simulink library "mylib"  (R2020a)
settings: Solver=VariableStepAuto  StartTime=0.0  StopTime=10.0  RelTol=1e-3
undefined symbols (not defined in the file): d_du_max_pu, dir_to_bus1, dir_to_bus_0L, dir_to_bus_2, dir_to_line1, dir_to_line_0L, dir_to_line_2, du_max_pu, du_ph_max_pu, Fi_0, Fi_T_H, Fi_T_L, Fi_T_M, I0_calc_0L, I0_comp_H, I0_comp_L, I0_comp_M, I0_max_0L, I2_max_2, I_diff1, I_diff2, I_diff3, I_diff4, I_diff5, I_diff_to, I_hight_CT1_G, I_hight_CT2_G, I_low_CT1, I_low_CT2, I_max1, I_max2, I_max3, I_max4, I_max5, I_min_sec_CT1, I_min_sec_CT2, I_unb, Iph_max_0L, Iph_max_2, jmp_in_zone, jmp_in_zone_0L, jmp_in_zone_2, K_dop, max_min1, only_K1_0L, only_K1_2, only_K2_0L, only_K2_2, only_K3_0L, only_K3_2, P_ctl_0, PQ_Fi_ctl_0, Q_ctl_0, S_set_0, set, set1, T_fast, T_I_ctl, T_off, T_on ... (+15)
libraries: $bdroot x184, powerlib_meascontrol x97
(part 12 of 14)

== system mylib/278_dzt_v1/diff_brake/calc_brake_Ia/cut_brake_1 ==
  Y_in : Inport
  I_max : Inport  Port=2
  I_diff_cur1 : Inport  Port=3
  I_max_cur1 : Inport  Port=4
  I_diff_cur2 : Inport  Port=5
  I_max_cur2 : Inport  Port=6
  I_diff_next : Inport  Port=7
  I_max_next : Inport  Port=8
  I_diff_to : Inport  Port=9
  1 : RelationalOperator  Operator=>  OutDataTypeStr=boolean  RndMeth=Simplest
  10 : Sum  Inputs=+-
  11 : Sum
  12 : Product
  13 : Sum
  {2,14..16,20} (5 alike) : Switch  Criteria=u2 > Threshold
  157 : Constant  Value=0
  17 : Logic  AllPortsSameDT=off  OutDataTypeStr=boolean
  18 : Logic  AllPortsSameDT=off  OutDataTypeStr=boolean
  19 : Logic  Operator=NOT  AllPortsSameDT=off  OutDataTypeStr=boolean
  3 : Product  Inputs=*/  RndMeth=Zero  SaturateOnIntegerOverflow=on
  4 : Product
  5 : Sum
  6 : RelationalOperator  Operator=<=  OutDataTypeStr=boolean  RndMeth=Simplest
  7 : RelationalOperator  Operator=>  OutDataTypeStr=boolean  RndMeth=Simplest
  8 : Logic  Operator=OR  AllPortsSameDT=off  OutDataTypeStr=boolean
  9 : RelationalOperator  Operator===  OutDataTypeStr=boolean  RndMeth=Simplest
  ADD_B : Subsystem
  ADD_K : Subsystem
  z_ch : Subsystem
  z_ch1 : Subsystem
  z_ch2 : Subsystem
  I_brake : Outport
  wires:
  20/1 -> 7/2, 6/2
  11/1 -> 20/1
  18/1 -> 20/2
  z_ch2/1(out) -> 18/1
  19/1 -> 18/2
  5/1 -> 2/1
  17/1 -> 2/2
  6/1 -> 17/2
  1/1 -> 17/1
  7/1 -> 15/2
  4/1 -> 5/1
  2/1 -> 15/3
  14/1 -> 15/1
  8/1 -> 16/2
  15/1 -> 16/3
  16/1 -> I_brake/1
  9/1 -> 19/1, 14/2
  13/1 -> 14/1
  ADD_B/1(out) -> 13/2, 5/2
  12/1 -> 13/1
  157/1 -> 9/2
  I_diff_to/1 -> 10/1, 14/3, 9/1
  3/1 -> 11/1
  10/1 -> 3/1
  ADD_K/1(out) -> 3/2, 12/1, 4/2
  I_max_next/1 -> z_ch2/2(in2)
  I_diff_next/1 -> z_ch2/1(in1)
  I_max_cur2/1 -> z_ch1/2(in2), ADD_B/2(X2), ADD_K/3(X2), 20/3
  I_diff_cur2/1 -> ADD_B/3(Y2), ADD_K/1(Y2), z_ch1/1(in1)
  I_max_cur1/1 -> ADD_B/4(X1), ADD_K/4(X1), 1/2, z_ch/2(in2), 11/2
  I_diff_cur1/1 -> z_ch/1(in1), ADD_B/1(Y1), ADD_K/2(Y1), 10/2
  z_ch1/1(out) -> 8/2
  z_ch/1(out) -> 8/1
  I_max/1 -> 1/1, 6/1, 4/1, 7/1, 12/2
  Y_in/1 -> 2/3, 16/1

== system mylib/278_dzt_v1/diff_brake/calc_brake_Ia/cut_brake_2 ==
  Y_in : Inport
  I_max : Inport  Port=2
  I_diff_cur1 : Inport  Port=3
  I_max_cur1 : Inport  Port=4
  I_diff_cur2 : Inport  Port=5
  I_max_cur2 : Inport  Port=6
  I_diff_next : Inport  Port=7
  I_max_next : Inport  Port=8
  I_diff_to : Inport  Port=9
  1 : RelationalOperator  Operator=>  OutDataTypeStr=boolean  RndMeth=Simplest
  10 : Sum  Inputs=+-
  11 : Sum
  12 : Product
  13 : Sum
  {2,14..16,20} (5 alike) : Switch  Criteria=u2 > Threshold
  157 : Constant  Value=0
  17 : Logic  AllPortsSameDT=off  OutDataTypeStr=boolean
  18 : Logic  AllPortsSameDT=off  OutDataTypeStr=boolean
  19 : Logic  Operator=NOT  AllPortsSameDT=off  OutDataTypeStr=boolean
  3 : Product  Inputs=*/  RndMeth=Zero  SaturateOnIntegerOverflow=on
  4 : Product
  5 : Sum
  6 : RelationalOperator  Operator=<=  OutDataTypeStr=boolean  RndMeth=Simplest
  7 : RelationalOperator  Operator=>  OutDataTypeStr=boolean  RndMeth=Simplest
  8 : Logic  Operator=OR  AllPortsSameDT=off  OutDataTypeStr=boolean
  9 : RelationalOperator  Operator===  OutDataTypeStr=boolean  RndMeth=Simplest
  ADD_B : Subsystem
  ADD_K : Subsystem
  z_ch : Subsystem
  z_ch1 : Subsystem
  z_ch2 : Subsystem
  I_brake : Outport
  wires:
  20/1 -> 7/2, 6/2
  11/1 -> 20/1
  18/1 -> 20/2
  z_ch2/1(out) -> 18/1
  19/1 -> 18/2
  5/1 -> 2/1
  17/1 -> 2/2
  6/1 -> 17/2
  1/1 -> 17/1
  7/1 -> 15/2
  4/1 -> 5/1
  2/1 -> 15/3
  14/1 -> 15/1
  8/1 -> 16/2
  15/1 -> 16/3
  16/1 -> I_brake/1
  9/1 -> 19/1, 14/2
  13/1 -> 14/1
  ADD_B/1(out) -> 13/2, 5/2
  12/1 -> 13/1
  157/1 -> 9/2
  I_diff_to/1 -> 10/1, 14/3, 9/1
  3/1 -> 11/1
  10/1 -> 3/1
  ADD_K/1(out) -> 3/2, 12/1, 4/2
  I_max_next/1 -> z_ch2/2(in2)
  I_diff_next/1 -> z_ch2/1(in1)
  I_max_cur2/1 -> z_ch1/2(in2), ADD_B/2(X2), ADD_K/3(X2), 20/3
  I_diff_cur2/1 -> ADD_B/3(Y2), ADD_K/1(Y2), z_ch1/1(in1)
  I_max_cur1/1 -> ADD_B/4(X1), ADD_K/4(X1), 1/2, z_ch/2(in2), 11/2
  I_diff_cur1/1 -> z_ch/1(in1), ADD_B/1(Y1), ADD_K/2(Y1), 10/2
  z_ch1/1(out) -> 8/2
  z_ch/1(out) -> 8/1
  I_max/1 -> 1/1, 6/1, 4/1, 7/1, 12/2
  Y_in/1 -> 2/3, 16/1

== system mylib/278_dzt_v1/diff_brake/calc_brake_Ia/cut_brake_3 ==
  Y_in : Inport
  I_max : Inport  Port=2
  I_diff_cur1 : Inport  Port=3
  I_max_cur1 : Inport  Port=4
  I_diff_cur2 : Inport  Port=5
  I_max_cur2 : Inport  Port=6
  I_diff_next : Inport  Port=7
  I_max_next : Inport  Port=8
  I_diff_to : Inport  Port=9
  1 : RelationalOperator  Operator=>  OutDataTypeStr=boolean  RndMeth=Simplest
  10 : Sum  Inputs=+-
  11 : Sum
  12 : Product
  13 : Sum
  {2,14..16,20} (5 alike) : Switch  Criteria=u2 > Threshold
  157 : Constant  Value=0
  17 : Logic  AllPortsSameDT=off  OutDataTypeStr=boolean
  18 : Logic  AllPortsSameDT=off  OutDataTypeStr=boolean
  19 : Logic  Operator=NOT  AllPortsSameDT=off  OutDataTypeStr=boolean
  3 : Product  Inputs=*/  RndMeth=Zero  SaturateOnIntegerOverflow=on
  4 : Product
  5 : Sum
  6 : RelationalOperator  Operator=<=  OutDataTypeStr=boolean  RndMeth=Simplest
  7 : RelationalOperator  Operator=>  OutDataTypeStr=boolean  RndMeth=Simplest
  8 : Logic  Operator=OR  AllPortsSameDT=off  OutDataTypeStr=boolean
  9 : RelationalOperator  Operator===  OutDataTypeStr=boolean  RndMeth=Simplest
  ADD_B : Subsystem
  ADD_K : Subsystem
  z_ch : Subsystem
  z_ch1 : Subsystem
  z_ch2 : Subsystem
  I_brake : Outport
  wires:
  20/1 -> 7/2, 6/2
  11/1 -> 20/1
  18/1 -> 20/2
  z_ch2/1(out) -> 18/1
  19/1 -> 18/2
  5/1 -> 2/1
  17/1 -> 2/2
  6/1 -> 17/2
  1/1 -> 17/1
  7/1 -> 15/2
  4/1 -> 5/1
  2/1 -> 15/3
  14/1 -> 15/1
  8/1 -> 16/2
  15/1 -> 16/3
  16/1 -> I_brake/1
  9/1 -> 19/1, 14/2
  13/1 -> 14/1
  ADD_B/1(out) -> 13/2, 5/2
  12/1 -> 13/1
  157/1 -> 9/2
  I_diff_to/1 -> 10/1, 14/3, 9/1
  3/1 -> 11/1
  10/1 -> 3/1
  ADD_K/1(out) -> 3/2, 12/1, 4/2
  I_max_next/1 -> z_ch2/2(in2)
  I_diff_next/1 -> z_ch2/1(in1)
  I_max_cur2/1 -> z_ch1/2(in2), ADD_B/2(X2), ADD_K/3(X2), 20/3
  I_diff_cur2/1 -> ADD_B/3(Y2), ADD_K/1(Y2), z_ch1/1(in1)
  I_max_cur1/1 -> ADD_B/4(X1), ADD_K/4(X1), 1/2, z_ch/2(in2), 11/2
  I_diff_cur1/1 -> z_ch/1(in1), ADD_B/1(Y1), ADD_K/2(Y1), 10/2
  z_ch1/1(out) -> 8/2
  z_ch/1(out) -> 8/1
  I_max/1 -> 1/1, 6/1, 4/1, 7/1, 12/2
  Y_in/1 -> 2/3, 16/1

== system mylib/278_dzt_v1/diff_brake/calc_brake_Ia/cut_brake_4 ==
  Y_in : Inport
  I_max : Inport  Port=2
  I_diff_cur1 : Inport  Port=3
  I_max_cur1 : Inport  Port=4
  I_diff_cur2 : Inport  Port=5
  I_max_cur2 : Inport  Port=6
  I_diff_next : Inport  Port=7
  I_max_next : Inport  Port=8
  I_diff_to : Inport  Port=9
  1 : RelationalOperator  Operator=>  OutDataTypeStr=boolean  RndMeth=Simplest
  10 : Sum  Inputs=+-
  11 : Sum
  12 : Product
  13 : Sum
  {2,14..16,20} (5 alike) : Switch  Criteria=u2 > Threshold
  157 : Constant  Value=0
  17 : Logic  AllPortsSameDT=off  OutDataTypeStr=boolean
  18 : Logic  AllPortsSameDT=off  OutDataTypeStr=boolean
  19 : Logic  Operator=NOT  AllPortsSameDT=off  OutDataTypeStr=boolean
  3 : Product  Inputs=*/  RndMeth=Zero  SaturateOnIntegerOverflow=on
  4 : Product
  5 : Sum
  6 : RelationalOperator  Operator=<=  OutDataTypeStr=boolean  RndMeth=Simplest
  7 : RelationalOperator  Operator=>  OutDataTypeStr=boolean  RndMeth=Simplest
  8 : Logic  Operator=OR  AllPortsSameDT=off  OutDataTypeStr=boolean
  9 : RelationalOperator  Operator===  OutDataTypeStr=boolean  RndMeth=Simplest
  ADD_B : Subsystem
  ADD_K : Subsystem
  z_ch : Subsystem
  z_ch1 : Subsystem
  z_ch2 : Subsystem
  I_brake : Outport
  wires:
  20/1 -> 7/2, 6/2
  11/1 -> 20/1
  18/1 -> 20/2
  z_ch2/1(out) -> 18/1
  19/1 -> 18/2
  5/1 -> 2/1
  17/1 -> 2/2
  6/1 -> 17/2
  1/1 -> 17/1
  7/1 -> 15/2
  4/1 -> 5/1
  2/1 -> 15/3
  14/1 -> 15/1
  8/1 -> 16/2
  15/1 -> 16/3
  16/1 -> I_brake/1
  9/1 -> 19/1, 14/2
  13/1 -> 14/1
  ADD_B/1(out) -> 13/2, 5/2
  12/1 -> 13/1
  157/1 -> 9/2
  I_diff_to/1 -> 10/1, 14/3, 9/1
  3/1 -> 11/1
  10/1 -> 3/1
  ADD_K/1(out) -> 3/2, 12/1, 4/2
  I_max_next/1 -> z_ch2/2(in2)
  I_diff_next/1 -> z_ch2/1(in1)
  I_max_cur2/1 -> z_ch1/2(in2), ADD_B/2(X2), ADD_K/3(X2), 20/3
  I_diff_cur2/1 -> ADD_B/3(Y2), ADD_K/1(Y2), z_ch1/1(in1)
  I_max_cur1/1 -> ADD_B/4(X1), ADD_K/4(X1), 1/2, z_ch/2(in2), 11/2
  I_diff_cur1/1 -> z_ch/1(in1), ADD_B/1(Y1), ADD_K/2(Y1), 10/2
  z_ch1/1(out) -> 8/2
  z_ch/1(out) -> 8/1
  I_max/1 -> 1/1, 6/1, 4/1, 7/1, 12/2
  Y_in/1 -> 2/3, 16/1

== system mylib/278_dzt_v1/diff_brake/calc_brake_Ib/cut_brake_1 ==
  Y_in : Inport
  I_max : Inport  Port=2
  I_diff_cur1 : Inport  Port=3
  I_max_cur1 : Inport  Port=4
  I_diff_cur2 : Inport  Port=5
  I_max_cur2 : Inport  Port=6
  I_diff_next : Inport  Port=7
  I_max_next : Inport  Port=8
  I_diff_to : Inport  Port=9
  1 : RelationalOperator  Operator=>  OutDataTypeStr=boolean  RndMeth=Simplest
  10 : Sum  Inputs=+-
  11 : Sum
  12 : Product
  13 : Sum
  {2,14..16,20} (5 alike) : Switch  Criteria=u2 > Threshold
  157 : Constant  Value=0
  17 : Logic  AllPortsSameDT=off  OutDataTypeStr=boolean
  18 : Logic  AllPortsSameDT=off  OutDataTypeStr=boolean
  19 : Logic  Operator=NOT  AllPortsSameDT=off  OutDataTypeStr=boolean
  3 : Product  Inputs=*/  RndMeth=Zero  SaturateOnIntegerOverflow=on
  4 : Product
  5 : Sum
  6 : RelationalOperator  Operator=<=  OutDataTypeStr=boolean  RndMeth=Simplest
  7 : RelationalOperator  Operator=>  OutDataTypeStr=boolean  RndMeth=Simplest
  8 : Logic  Operator=OR  AllPortsSameDT=off  OutDataTypeStr=boolean
  9 : RelationalOperator  Operator===  OutDataTypeStr=boolean  RndMeth=Simplest
  ADD_B : Subsystem
  ADD_K : Subsystem
  z_ch : Subsystem
  z_ch1 : Subsystem
  z_ch2 : Subsystem
  I_brake : Outport
  wires:
  20/1 -> 7/2, 6/2
  11/1 -> 20/1
  18/1 -> 20/2
  z_ch2/1(out) -> 18/1
  19/1 -> 18/2
  5/1 -> 2/1
  17/1 -> 2/2
  6/1 -> 17/2
  1/1 -> 17/1
  7/1 -> 15/2
  4/1 -> 5/1
  2/1 -> 15/3
  14/1 -> 15/1
  8/1 -> 16/2
  15/1 -> 16/3
  16/1 -> I_brake/1
  9/1 -> 19/1, 14/2
  13/1 -> 14/1
  ADD_B/1(out) -> 13/2, 5/2
  12/1 -> 13/1
  157/1 -> 9/2
  I_diff_to/1 -> 10/1, 14/3, 9/1
  3/1 -> 11/1
  10/1 -> 3/1
  ADD_K/1(out) -> 3/2, 12/1, 4/2
  I_max_next/1 -> z_ch2/2(in2)
  I_diff_next/1 -> z_ch2/1(in1)
  I_max_cur2/1 -> z_ch1/2(in2), ADD_B/2(X2), ADD_K/3(X2), 20/3
  I_diff_cur2/1 -> ADD_B/3(Y2), ADD_K/1(Y2), z_ch1/1(in1)
  I_max_cur1/1 -> ADD_B/4(X1), ADD_K/4(X1), 1/2, z_ch/2(in2), 11/2
  I_diff_cur1/1 -> z_ch/1(in1), ADD_B/1(Y1), ADD_K/2(Y1), 10/2
  z_ch1/1(out) -> 8/2
  z_ch/1(out) -> 8/1
  I_max/1 -> 1/1, 6/1, 4/1, 7/1, 12/2
  Y_in/1 -> 2/3, 16/1

== system mylib/278_dzt_v1/diff_brake/calc_brake_Ib/cut_brake_2 ==
  Y_in : Inport
  I_max : Inport  Port=2
  I_diff_cur1 : Inport  Port=3
  I_max_cur1 : Inport  Port=4
  I_diff_cur2 : Inport  Port=5
  I_max_cur2 : Inport  Port=6
  I_diff_next : Inport  Port=7
  I_max_next : Inport  Port=8
  I_diff_to : Inport  Port=9
  1 : RelationalOperator  Operator=>  OutDataTypeStr=boolean  RndMeth=Simplest
  10 : Sum  Inputs=+-
  11 : Sum
  12 : Product
  13 : Sum
  {2,14..16,20} (5 alike) : Switch  Criteria=u2 > Threshold
  157 : Constant  Value=0
  17 : Logic  AllPortsSameDT=off  OutDataTypeStr=boolean
  18 : Logic  AllPortsSameDT=off  OutDataTypeStr=boolean
  19 : Logic  Operator=NOT  AllPortsSameDT=off  OutDataTypeStr=boolean
  3 : Product  Inputs=*/  RndMeth=Zero  SaturateOnIntegerOverflow=on
  4 : Product
  5 : Sum
  6 : RelationalOperator  Operator=<=  OutDataTypeStr=boolean  RndMeth=Simplest
  7 : RelationalOperator  Operator=>  OutDataTypeStr=boolean  RndMeth=Simplest
  8 : Logic  Operator=OR  AllPortsSameDT=off  OutDataTypeStr=boolean
  9 : RelationalOperator  Operator===  OutDataTypeStr=boolean  RndMeth=Simplest
  ADD_B : Subsystem
  ADD_K : Subsystem
  z_ch : Subsystem
  z_ch1 : Subsystem
  z_ch2 : Subsystem
  I_brake : Outport
  wires:
  20/1 -> 7/2, 6/2
  11/1 -> 20/1
  18/1 -> 20/2
  z_ch2/1(out) -> 18/1
  19/1 -> 18/2
  5/1 -> 2/1
  17/1 -> 2/2
  6/1 -> 17/2
  1/1 -> 17/1
  7/1 -> 15/2
  4/1 -> 5/1
  2/1 -> 15/3
  14/1 -> 15/1
  8/1 -> 16/2
  15/1 -> 16/3
  16/1 -> I_brake/1
  9/1 -> 19/1, 14/2
  13/1 -> 14/1
  ADD_B/1(out) -> 13/2, 5/2
  12/1 -> 13/1
  157/1 -> 9/2
  I_diff_to/1 -> 10/1, 14/3, 9/1
  3/1 -> 11/1
  10/1 -> 3/1
  ADD_K/1(out) -> 3/2, 12/1, 4/2
  I_max_next/1 -> z_ch2/2(in2)
  I_diff_next/1 -> z_ch2/1(in1)
  I_max_cur2/1 -> z_ch1/2(in2), ADD_B/2(X2), ADD_K/3(X2), 20/3
  I_diff_cur2/1 -> ADD_B/3(Y2), ADD_K/1(Y2), z_ch1/1(in1)
  I_max_cur1/1 -> ADD_B/4(X1), ADD_K/4(X1), 1/2, z_ch/2(in2), 11/2
  I_diff_cur1/1 -> z_ch/1(in1), ADD_B/1(Y1), ADD_K/2(Y1), 10/2
  z_ch1/1(out) -> 8/2
  z_ch/1(out) -> 8/1
  I_max/1 -> 1/1, 6/1, 4/1, 7/1, 12/2
  Y_in/1 -> 2/3, 16/1

== system mylib/278_dzt_v1/diff_brake/calc_brake_Ib/cut_brake_3 ==
  Y_in : Inport
  I_max : Inport  Port=2
  I_diff_cur1 : Inport  Port=3
  I_max_cur1 : Inport  Port=4
  I_diff_cur2 : Inport  Port=5
  I_max_cur2 : Inport  Port=6
  I_diff_next : Inport  Port=7
  I_max_next : Inport  Port=8
  I_diff_to : Inport  Port=9
  1 : RelationalOperator  Operator=>  OutDataTypeStr=boolean  RndMeth=Simplest
  10 : Sum  Inputs=+-
  11 : Sum
  12 : Product
  13 : Sum
  {2,14..16,20} (5 alike) : Switch  Criteria=u2 > Threshold
  157 : Constant  Value=0
  17 : Logic  AllPortsSameDT=off  OutDataTypeStr=boolean
  18 : Logic  AllPortsSameDT=off  OutDataTypeStr=boolean
  19 : Logic  Operator=NOT  AllPortsSameDT=off  OutDataTypeStr=boolean
  3 : Product  Inputs=*/  RndMeth=Zero  SaturateOnIntegerOverflow=on
  4 : Product
  5 : Sum
  6 : RelationalOperator  Operator=<=  OutDataTypeStr=boolean  RndMeth=Simplest
  7 : RelationalOperator  Operator=>  OutDataTypeStr=boolean  RndMeth=Simplest
  8 : Logic  Operator=OR  AllPortsSameDT=off  OutDataTypeStr=boolean
  9 : RelationalOperator  Operator===  OutDataTypeStr=boolean  RndMeth=Simplest
  ADD_B : Subsystem
  ADD_K : Subsystem
  z_ch : Subsystem
  z_ch1 : Subsystem
  z_ch2 : Subsystem
  I_brake : Outport
  wires:
  20/1 -> 7/2, 6/2
  11/1 -> 20/1
  18/1 -> 20/2
  z_ch2/1(out) -> 18/1
  19/1 -> 18/2
  5/1 -> 2/1
  17/1 -> 2/2
  6/1 -> 17/2
  1/1 -> 17/1
  7/1 -> 15/2
  4/1 -> 5/1
  2/1 -> 15/3
  14/1 -> 15/1
  8/1 -> 16/2
  15/1 -> 16/3
  16/1 -> I_brake/1
  9/1 -> 19/1, 14/2
  13/1 -> 14/1
  ADD_B/1(out) -> 13/2, 5/2
  12/1 -> 13/1
  157/1 -> 9/2
  I_diff_to/1 -> 10/1, 14/3, 9/1
  3/1 -> 11/1
  10/1 -> 3/1
  ADD_K/1(out) -> 3/2, 12/1, 4/2
  I_max_next/1 -> z_ch2/2(in2)
  I_diff_next/1 -> z_ch2/1(in1)
  I_max_cur2/1 -> z_ch1/2(in2), ADD_B/2(X2), ADD_K/3(X2), 20/3
  I_diff_cur2/1 -> ADD_B/3(Y2), ADD_K/1(Y2), z_ch1/1(in1)
  I_max_cur1/1 -> ADD_B/4(X1), ADD_K/4(X1), 1/2, z_ch/2(in2), 11/2
  I_diff_cur1/1 -> z_ch/1(in1), ADD_B/1(Y1), ADD_K/2(Y1), 10/2
  z_ch1/1(out) -> 8/2
  z_ch/1(out) -> 8/1
  I_max/1 -> 1/1, 6/1, 4/1, 7/1, 12/2
  Y_in/1 -> 2/3, 16/1

== system mylib/278_dzt_v1/diff_brake/calc_brake_Ib/cut_brake_4 ==
  Y_in : Inport
  I_max : Inport  Port=2
  I_diff_cur1 : Inport  Port=3
  I_max_cur1 : Inport  Port=4
  I_diff_cur2 : Inport  Port=5
  I_max_cur2 : Inport  Port=6
  I_diff_next : Inport  Port=7
  I_max_next : Inport  Port=8
  I_diff_to : Inport  Port=9
  1 : RelationalOperator  Operator=>  OutDataTypeStr=boolean  RndMeth=Simplest
  10 : Sum  Inputs=+-
  11 : Sum
  12 : Product
  13 : Sum
  {2,14..16,20} (5 alike) : Switch  Criteria=u2 > Threshold
  157 : Constant  Value=0
  17 : Logic  AllPortsSameDT=off  OutDataTypeStr=boolean
  18 : Logic  AllPortsSameDT=off  OutDataTypeStr=boolean
  19 : Logic  Operator=NOT  AllPortsSameDT=off  OutDataTypeStr=boolean
  3 : Product  Inputs=*/  RndMeth=Zero  SaturateOnIntegerOverflow=on
  4 : Product
  5 : Sum
  6 : RelationalOperator  Operator=<=  OutDataTypeStr=boolean  RndMeth=Simplest
  7 : RelationalOperator  Operator=>  OutDataTypeStr=boolean  RndMeth=Simplest
  8 : Logic  Operator=OR  AllPortsSameDT=off  OutDataTypeStr=boolean
  9 : RelationalOperator  Operator===  OutDataTypeStr=boolean  RndMeth=Simplest
  ADD_B : Subsystem
  ADD_K : Subsystem
  z_ch : Subsystem
  z_ch1 : Subsystem
  z_ch2 : Subsystem
  I_brake : Outport
  wires:
  20/1 -> 7/2, 6/2
  11/1 -> 20/1
  18/1 -> 20/2
  z_ch2/1(out) -> 18/1
  19/1 -> 18/2
  5/1 -> 2/1
  17/1 -> 2/2
  6/1 -> 17/2
  1/1 -> 17/1
  7/1 -> 15/2
  4/1 -> 5/1
  2/1 -> 15/3
  14/1 -> 15/1
  8/1 -> 16/2
  15/1 -> 16/3
  16/1 -> I_brake/1
  9/1 -> 19/1, 14/2
  13/1 -> 14/1
  ADD_B/1(out) -> 13/2, 5/2
  12/1 -> 13/1
  157/1 -> 9/2
  I_diff_to/1 -> 10/1, 14/3, 9/1
  3/1 -> 11/1
  10/1 -> 3/1
  ADD_K/1(out) -> 3/2, 12/1, 4/2
  I_max_next/1 -> z_ch2/2(in2)
  I_diff_next/1 -> z_ch2/1(in1)
  I_max_cur2/1 -> z_ch1/2(in2), ADD_B/2(X2), ADD_K/3(X2), 20/3
  I_diff_cur2/1 -> ADD_B/3(Y2), ADD_K/1(Y2), z_ch1/1(in1)
  I_max_cur1/1 -> ADD_B/4(X1), ADD_K/4(X1), 1/2, z_ch/2(in2), 11/2
  I_diff_cur1/1 -> z_ch/1(in1), ADD_B/1(Y1), ADD_K/2(Y1), 10/2
  z_ch1/1(out) -> 8/2
  z_ch/1(out) -> 8/1
  I_max/1 -> 1/1, 6/1, 4/1, 7/1, 12/2
  Y_in/1 -> 2/3, 16/1

== system mylib/278_dzt_v1/diff_brake/calc_brake_Ic/cut_brake_1 ==
  Y_in : Inport
  I_max : Inport  Port=2
  I_diff_cur1 : Inport  Port=3
  I_max_cur1 : Inport  Port=4
  I_diff_cur2 : Inport  Port=5
  I_max_cur2 : Inport  Port=6
  I_diff_next : Inport  Port=7
  I_max_next : Inport  Port=8
  I_diff_to : Inport  Port=9
  1 : RelationalOperator  Operator=>  OutDataTypeStr=boolean  RndMeth=Simplest
  10 : Sum  Inputs=+-
  11 : Sum
  12 : Product
  13 : Sum
  {2,14..16,20} (5 alike) : Switch  Criteria=u2 > Threshold
  157 : Constant  Value=0
  17 : Logic  AllPortsSameDT=off  OutDataTypeStr=boolean
  18 : Logic  AllPortsSameDT=off  OutDataTypeStr=boolean
  19 : Logic  Operator=NOT  AllPortsSameDT=off  OutDataTypeStr=boolean
  3 : Product  Inputs=*/  RndMeth=Zero  SaturateOnIntegerOverflow=on
  4 : Product
  5 : Sum
  6 : RelationalOperator  Operator=<=  OutDataTypeStr=boolean  RndMeth=Simplest
  7 : RelationalOperator  Operator=>  OutDataTypeStr=boolean  RndMeth=Simplest
  8 : Logic  Operator=OR  AllPortsSameDT=off  OutDataTypeStr=boolean
  9 : RelationalOperator  Operator===  OutDataTypeStr=boolean  RndMeth=Simplest
  ADD_B : Subsystem
  ADD_K : Subsystem
  z_ch : Subsystem
  z_ch1 : Subsystem
  z_ch2 : Subsystem
  I_brake : Outport
  wires:
  20/1 -> 7/2, 6/2
  11/1 -> 20/1
  18/1 -> 20/2
  z_ch2/1(out) -> 18/1
  19/1 -> 18/2
  5/1 -> 2/1
  17/1 -> 2/2
  6/1 -> 17/2
  1/1 -> 17/1
  7/1 -> 15/2
  4/1 -> 5/1
  2/1 -> 15/3
  14/1 -> 15/1
  8/1 -> 16/2
  15/1 -> 16/3
  16/1 -> I_brake/1
  9/1 -> 19/1, 14/2
  13/1 -> 14/1
  ADD_B/1(out) -> 13/2, 5/2
  12/1 -> 13/1
  157/1 -> 9/2
  I_diff_to/1 -> 10/1, 14/3, 9/1
  3/1 -> 11/1
  10/1 -> 3/1
  ADD_K/1(out) -> 3/2, 12/1, 4/2
  I_max_next/1 -> z_ch2/2(in2)
  I_diff_next/1 -> z_ch2/1(in1)
  I_max_cur2/1 -> z_ch1/2(in2), ADD_B/2(X2), ADD_K/3(X2), 20/3
  I_diff_cur2/1 -> ADD_B/3(Y2), ADD_K/1(Y2), z_ch1/1(in1)
  I_max_cur1/1 -> ADD_B/4(X1), ADD_K/4(X1), 1/2, z_ch/2(in2), 11/2
  I_diff_cur1/1 -> z_ch/1(in1), ADD_B/1(Y1), ADD_K/2(Y1), 10/2
  z_ch1/1(out) -> 8/2
  z_ch/1(out) -> 8/1
  I_max/1 -> 1/1, 6/1, 4/1, 7/1, 12/2
  Y_in/1 -> 2/3, 16/1

== system mylib/278_dzt_v1/diff_brake/calc_brake_Ic/cut_brake_2 ==
  Y_in : Inport
  I_max : Inport  Port=2
  I_diff_cur1 : Inport  Port=3
  I_max_cur1 : Inport  Port=4
  I_diff_cur2 : Inport  Port=5
  I_max_cur2 : Inport  Port=6
  I_diff_next : Inport  Port=7
  I_max_next : Inport  Port=8
  I_diff_to : Inport  Port=9
  1 : RelationalOperator  Operator=>  OutDataTypeStr=boolean  RndMeth=Simplest
  10 : Sum  Inputs=+-
  11 : Sum
  12 : Product
  13 : Sum
  {2,14..16,20} (5 alike) : Switch  Criteria=u2 > Threshold
  157 : Constant  Value=0
  17 : Logic  AllPortsSameDT=off  OutDataTypeStr=boolean
  18 : Logic  AllPortsSameDT=off  OutDataTypeStr=boolean
  19 : Logic  Operator=NOT  AllPortsSameDT=off  OutDataTypeStr=boolean
  3 : Product  Inputs=*/  RndMeth=Zero  SaturateOnIntegerOverflow=on
  4 : Product
  5 : Sum
  6 : RelationalOperator  Operator=<=  OutDataTypeStr=boolean  RndMeth=Simplest
  7 : RelationalOperator  Operator=>  OutDataTypeStr=boolean  RndMeth=Simplest
  8 : Logic  Operator=OR  AllPortsSameDT=off  OutDataTypeStr=boolean
  9 : RelationalOperator  Operator===  OutDataTypeStr=boolean  RndMeth=Simplest
  ADD_B : Subsystem
  ADD_K : Subsystem
  z_ch : Subsystem
  z_ch1 : Subsystem
  z_ch2 : Subsystem
  I_brake : Outport
  wires:
  20/1 -> 7/2, 6/2
  11/1 -> 20/1
  18/1 -> 20/2
  z_ch2/1(out) -> 18/1
  19/1 -> 18/2
  5/1 -> 2/1
  17/1 -> 2/2
  6/1 -> 17/2
  1/1 -> 17/1
  7/1 -> 15/2
  4/1 -> 5/1
  2/1 -> 15/3
  14/1 -> 15/1
  8/1 -> 16/2
  15/1 -> 16/3
  16/1 -> I_brake/1
  9/1 -> 19/1, 14/2
  13/1 -> 14/1
  ADD_B/1(out) -> 13/2, 5/2
  12/1 -> 13/1
  157/1 -> 9/2
  I_diff_to/1 -> 10/1, 14/3, 9/1
  3/1 -> 11/1
  10/1 -> 3/1
  ADD_K/1(out) -> 3/2, 12/1, 4/2
  I_max_next/1 -> z_ch2/2(in2)
  I_diff_next/1 -> z_ch2/1(in1)
  I_max_cur2/1 -> z_ch1/2(in2), ADD_B/2(X2), ADD_K/3(X2), 20/3
  I_diff_cur2/1 -> ADD_B/3(Y2), ADD_K/1(Y2), z_ch1/1(in1)
  I_max_cur1/1 -> ADD_B/4(X1), ADD_K/4(X1), 1/2, z_ch/2(in2), 11/2
  I_diff_cur1/1 -> z_ch/1(in1), ADD_B/1(Y1), ADD_K/2(Y1), 10/2
  z_ch1/1(out) -> 8/2
  z_ch/1(out) -> 8/1
  I_max/1 -> 1/1, 6/1, 4/1, 7/1, 12/2
  Y_in/1 -> 2/3, 16/1

== system mylib/278_dzt_v1/diff_brake/calc_brake_Ic/cut_brake_3 ==
  Y_in : Inport
  I_max : Inport  Port=2
  I_diff_cur1 : Inport  Port=3
  I_max_cur1 : Inport  Port=4
  I_diff_cur2 : Inport  Port=5
  I_max_cur2 : Inport  Port=6
  I_diff_next : Inport  Port=7
  I_max_next : Inport  Port=8
  I_diff_to : Inport  Port=9
  1 : RelationalOperator  Operator=>  OutDataTypeStr=boolean  RndMeth=Simplest
  10 : Sum  Inputs=+-
  11 : Sum
  12 : Product
  13 : Sum
  {2,14..16,20} (5 alike) : Switch  Criteria=u2 > Threshold
  157 : Constant  Value=0
  17 : Logic  AllPortsSameDT=off  OutDataTypeStr=boolean
  18 : Logic  AllPortsSameDT=off  OutDataTypeStr=boolean
  19 : Logic  Operator=NOT  AllPortsSameDT=off  OutDataTypeStr=boolean
  3 : Product  Inputs=*/  RndMeth=Zero  SaturateOnIntegerOverflow=on
  4 : Product
  5 : Sum
  6 : RelationalOperator  Operator=<=  OutDataTypeStr=boolean  RndMeth=Simplest
  7 : RelationalOperator  Operator=>  OutDataTypeStr=boolean  RndMeth=Simplest
  8 : Logic  Operator=OR  AllPortsSameDT=off  OutDataTypeStr=boolean
  9 : RelationalOperator  Operator===  OutDataTypeStr=boolean  RndMeth=Simplest
  ADD_B : Subsystem
  ADD_K : Subsystem
  z_ch : Subsystem
  z_ch1 : Subsystem
  z_ch2 : Subsystem
  I_brake : Outport
  wires:
  20/1 -> 7/2, 6/2
  11/1 -> 20/1
  18/1 -> 20/2
  z_ch2/1(out) -> 18/1
  19/1 -> 18/2
  5/1 -> 2/1
  17/1 -> 2/2
  6/1 -> 17/2
  1/1 -> 17/1
  7/1 -> 15/2
  4/1 -> 5/1
  2/1 -> 15/3
  14/1 -> 15/1
  8/1 -> 16/2
  15/1 -> 16/3
  16/1 -> I_brake/1
  9/1 -> 19/1, 14/2
  13/1 -> 14/1
  ADD_B/1(out) -> 13/2, 5/2
  12/1 -> 13/1
  157/1 -> 9/2
  I_diff_to/1 -> 10/1, 14/3, 9/1
  3/1 -> 11/1
  10/1 -> 3/1
  ADD_K/1(out) -> 3/2, 12/1, 4/2
  I_max_next/1 -> z_ch2/2(in2)
  I_diff_next/1 -> z_ch2/1(in1)
  I_max_cur2/1 -> z_ch1/2(in2), ADD_B/2(X2), ADD_K/3(X2), 20/3
  I_diff_cur2/1 -> ADD_B/3(Y2), ADD_K/1(Y2), z_ch1/1(in1)
  I_max_cur1/1 -> ADD_B/4(X1), ADD_K/4(X1), 1/2, z_ch/2(in2), 11/2
  I_diff_cur1/1 -> z_ch/1(in1), ADD_B/1(Y1), ADD_K/2(Y1), 10/2
  z_ch1/1(out) -> 8/2
  z_ch/1(out) -> 8/1
  I_max/1 -> 1/1, 6/1, 4/1, 7/1, 12/2
  Y_in/1 -> 2/3, 16/1

== system mylib/278_dzt_v1/diff_brake/calc_brake_Ic/cut_brake_4 ==
  Y_in : Inport
  I_max : Inport  Port=2
  I_diff_cur1 : Inport  Port=3
  I_max_cur1 : Inport  Port=4
  I_diff_cur2 : Inport  Port=5
  I_max_cur2 : Inport  Port=6
  I_diff_next : Inport  Port=7
  I_max_next : Inport  Port=8
  I_diff_to : Inport  Port=9
  1 : RelationalOperator  Operator=>  OutDataTypeStr=boolean  RndMeth=Simplest
  10 : Sum  Inputs=+-
  11 : Sum
  12 : Product
  13 : Sum
  {2,14..16,20} (5 alike) : Switch  Criteria=u2 > Threshold
  157 : Constant  Value=0
  17 : Logic  AllPortsSameDT=off  OutDataTypeStr=boolean
  18 : Logic  AllPortsSameDT=off  OutDataTypeStr=boolean
  19 : Logic  Operator=NOT  AllPortsSameDT=off  OutDataTypeStr=boolean
  3 : Product  Inputs=*/  RndMeth=Zero  SaturateOnIntegerOverflow=on
  4 : Product
  5 : Sum
  6 : RelationalOperator  Operator=<=  OutDataTypeStr=boolean  RndMeth=Simplest
  7 : RelationalOperator  Operator=>  OutDataTypeStr=boolean  RndMeth=Simplest
  8 : Logic  Operator=OR  AllPortsSameDT=off  OutDataTypeStr=boolean
  9 : RelationalOperator  Operator===  OutDataTypeStr=boolean  RndMeth=Simplest
  ADD_B : Subsystem
  ADD_K : Subsystem
  z_ch : Subsystem
  z_ch1 : Subsystem
  z_ch2 : Subsystem
  I_brake : Outport
  wires:
  20/1 -> 7/2, 6/2
  11/1 -> 20/1
  18/1 -> 20/2
  z_ch2/1(out) -> 18/1
  19/1 -> 18/2
  5/1 -> 2/1
  17/1 -> 2/2
  6/1 -> 17/2
  1/1 -> 17/1
  7/1 -> 15/2
  4/1 -> 5/1
  2/1 -> 15/3
  14/1 -> 15/1
  8/1 -> 16/2
  15/1 -> 16/3
  16/1 -> I_brake/1
  9/1 -> 19/1, 14/2
  13/1 -> 14/1
  ADD_B/1(out) -> 13/2, 5/2
  12/1 -> 13/1
  157/1 -> 9/2
  I_diff_to/1 -> 10/1, 14/3, 9/1
  3/1 -> 11/1
  10/1 -> 3/1
  ADD_K/1(out) -> 3/2, 12/1, 4/2
  I_max_next/1 -> z_ch2/2(in2)
  I_diff_next/1 -> z_ch2/1(in1)
  I_max_cur2/1 -> z_ch1/2(in2), ADD_B/2(X2), ADD_K/3(X2), 20/3
  I_diff_cur2/1 -> ADD_B/3(Y2), ADD_K/1(Y2), z_ch1/1(in1)
  I_max_cur1/1 -> ADD_B/4(X1), ADD_K/4(X1), 1/2, z_ch/2(in2), 11/2
  I_diff_cur1/1 -> z_ch/1(in1), ADD_B/1(Y1), ADD_K/2(Y1), 10/2
  z_ch1/1(out) -> 8/2
  z_ch/1(out) -> 8/1
  I_max/1 -> 1/1, 6/1, 4/1, 7/1, 12/2
  Y_in/1 -> 2/3, 16/1

== system mylib/278_dzt_v1/diff_trans_calc_H/Ia_calc/orto_MUL_orto ==
  F1re : Inport
  F1im : Inport  Port=2
  F2re : Inport  Port=3
  F2im : Inport  Port=4
  1 : Sum  Inputs=+-
  {2..5} (4 alike) : Product
  6 : Sum
  Fre : Outport
  Fim : Outport  Port=2
  wires:
  F2re/1 -> 4/2, 2/2
  F1im/1 -> 3/1, 4/1
  F2im/1 -> 3/2, 5/2
  5/1 -> 6/2
  4/1 -> 6/1
  3/1 -> 1/2
  2/1 -> 1/1
  6/1 -> Fim/1
  1/1 -> Fre/1
  F1re/1 -> 2/1, 5/1

== system mylib/278_dzt_v1/diff_trans_calc_H/Ia_calc/orto_to_arg ==
  re : Inport
  im : Inport  Port=2
  1 : Sum
  11 : Product  Inputs=*/  RndMeth=Zero  SaturateOnIntegerOverflow=on
  154 : Constant  Value=-1
  2 : Product
  3 : Switch  Criteria=u2 > Threshold
  4 : Sqrt  SaturateOnIntegerOverflow=on
  5 : Trigonometry  Operator=acos
  6 : Product
  7 : RelationalOperator  Operator=>  OutDataTypeStr=boolean  RndMeth=Simplest
  8 : Constant  Value=0
  9 : Product
  arg : Outport
  wires:
  4/1 -> 11/2
  11/1 -> 5/1
  2/1 -> 1/1
  6/1 -> 1/2
  1/1 -> 4/1
  5/1 -> 9/1, 3/1
  154/1 -> 9/2
  7/1 -> 3/2
  9/1 -> 3/3
  8/1 -> 7/2
  re/1 -> 2/1, 11/1, 2/2
  im/1 -> 6/1, 6/2, 7/1
  3/1 -> arg/1

== system mylib/278_dzt_v1/diff_trans_calc_H/Ia_diff_calc/module1 ==
  Re : Inport
  Im : Inport  Port=2
  1 : Product  Inputs=**
  2 : Sum
  3 : Product  Inputs=**
  4 : Sqrt  SaturateOnIntegerOverflow=on
  Module : Outport
  wires:
  Re/1 -> 1/1, 1/2
  2/1 -> 4/1
  4/1 -> Module/1
  Im/1 -> 3/2, 3/1
  1/1 -> 2/1
  3/1 -> 2/2

== system mylib/278_dzt_v1/diff_trans_calc_H/Ia_diff_calc/module2 ==
  Re : Inport
  Im : Inport  Port=2
  1 : Product  Inputs=**
  2 : Sum
  3 : Product  Inputs=**
  4 : Sqrt  SaturateOnIntegerOverflow=on
  Module : Outport
  wires:
  Re/1 -> 1/1, 1/2
  2/1 -> 4/1
  4/1 -> Module/1
  Im/1 -> 3/2, 3/1
  1/1 -> 2/1
  3/1 -> 2/2

== system mylib/278_dzt_v1/diff_trans_calc_H/Ib_calc/orto_MUL_orto ==
  F1re : Inport
  F1im : Inport  Port=2
  F2re : Inport  Port=3
  F2im : Inport  Port=4
  1 : Sum  Inputs=+-
  {2..5} (4 alike) : Product
  6 : Sum
  Fre : Outport
  Fim : Outport  Port=2
  wires:
  F2re/1 -> 4/2, 2/2
  F1im/1 -> 3/1, 4/1
  F2im/1 -> 3/2, 5/2
  5/1 -> 6/2
  4/1 -> 6/1
  3/1 -> 1/2
  2/1 -> 1/1
  6/1 -> Fim/1
  1/1 -> Fre/1
  F1re/1 -> 2/1, 5/1

== system mylib/278_dzt_v1/diff_trans_calc_H/Ib_calc/orto_to_arg ==
  re : Inport
  im : Inport  Port=2
  1 : Sum
  11 : Product  Inputs=*/  RndMeth=Zero  SaturateOnIntegerOverflow=on
  154 : Constant  Value=-1
  2 : Product
  3 : Switch  Criteria=u2 > Threshold
  4 : Sqrt  SaturateOnIntegerOverflow=on
  5 : Trigonometry  Operator=acos
  6 : Product
  7 : RelationalOperator  Operator=>  OutDataTypeStr=boolean  RndMeth=Simplest
  8 : Constant  Value=0
  9 : Product
  arg : Outport
  wires:
  4/1 -> 11/2
  11/1 -> 5/1
  2/1 -> 1/1
  6/1 -> 1/2
  1/1 -> 4/1
  5/1 -> 9/1, 3/1
  154/1 -> 9/2
  7/1 -> 3/2
  9/1 -> 3/3
  8/1 -> 7/2
  re/1 -> 2/1, 11/1, 2/2
  im/1 -> 6/1, 6/2, 7/1
  3/1 -> arg/1

== system mylib/278_dzt_v1/diff_trans_calc_H/Ib_diff_calc/module1 ==
  Re : Inport
  Im : Inport  Port=2
  1 : Product  Inputs=**
  2 : Sum
  3 : Product  Inputs=**
  4 : Sqrt  SaturateOnIntegerOverflow=on
  Module : Outport
  wires:
  Re/1 -> 1/1, 1/2
  2/1 -> 4/1
  4/1 -> Module/1
  Im/1 -> 3/2, 3/1
  1/1 -> 2/1
  3/1 -> 2/2

== system mylib/278_dzt_v1/diff_trans_calc_H/Ib_diff_calc/module2 ==
  Re : Inport
  Im : Inport  Port=2
  1 : Product  Inputs=**
  2 : Sum
  3 : Product  Inputs=**
  4 : Sqrt  SaturateOnIntegerOverflow=on
  Module : Outport
  wires:
  Re/1 -> 1/1, 1/2
  2/1 -> 4/1
  4/1 -> Module/1
  Im/1 -> 3/2, 3/1
  1/1 -> 2/1
  3/1 -> 2/2

== system mylib/278_dzt_v1/diff_trans_calc_H/Ic_calc/orto_MUL_orto ==
  F1re : Inport
  F1im : Inport  Port=2
  F2re : Inport  Port=3
  F2im : Inport  Port=4
  1 : Sum  Inputs=+-
  {2..5} (4 alike) : Product
  6 : Sum
  Fre : Outport
  Fim : Outport  Port=2
  wires:
  F2re/1 -> 4/2, 2/2
  F1im/1 -> 3/1, 4/1
  F2im/1 -> 3/2, 5/2
  5/1 -> 6/2
  4/1 -> 6/1
  3/1 -> 1/2
  2/1 -> 1/1
  6/1 -> Fim/1
  1/1 -> Fre/1
  F1re/1 -> 2/1, 5/1

== system mylib/278_dzt_v1/diff_trans_calc_H/Ic_calc/orto_to_arg ==
  re : Inport
  im : Inport  Port=2
  1 : Sum
  11 : Product  Inputs=*/  RndMeth=Zero  SaturateOnIntegerOverflow=on
  154 : Constant  Value=-1
  2 : Product
  3 : Switch  Criteria=u2 > Threshold
  4 : Sqrt  SaturateOnIntegerOverflow=on
  5 : Trigonometry  Operator=acos
  6 : Product
  7 : RelationalOperator  Operator=>  OutDataTypeStr=boolean  RndMeth=Simplest
  8 : Constant  Value=0
  9 : Product
  arg : Outport
  wires:
  4/1 -> 11/2
  11/1 -> 5/1
  2/1 -> 1/1
  6/1 -> 1/2
  1/1 -> 4/1
  5/1 -> 9/1, 3/1
  154/1 -> 9/2
  7/1 -> 3/2
  9/1 -> 3/3
  8/1 -> 7/2
  re/1 -> 2/1, 11/1, 2/2
  im/1 -> 6/1, 6/2, 7/1
  3/1 -> arg/1

== system mylib/278_dzt_v1/diff_trans_calc_H/Ic_diff_calc/module1 ==
  Re : Inport
  Im : Inport  Port=2
  1 : Product  Inputs=**
  2 : Sum
  3 : Product  Inputs=**
  4 : Sqrt  SaturateOnIntegerOverflow=on
  Module : Outport
  wires:
  Re/1 -> 1/1, 1/2
  2/1 -> 4/1
  4/1 -> Module/1
  Im/1 -> 3/2, 3/1
  1/1 -> 2/1
  3/1 -> 2/2

== system mylib/278_dzt_v1/diff_trans_calc_H/Ic_diff_calc/module2 ==
  Re : Inport
  Im : Inport  Port=2
  1 : Product  Inputs=**
  2 : Sum
  3 : Product  Inputs=**
  4 : Sqrt  SaturateOnIntegerOverflow=on
  Module : Outport
  wires:
  Re/1 -> 1/1, 1/2
  2/1 -> 4/1
  4/1 -> Module/1
  Im/1 -> 3/2, 3/1
  1/1 -> 2/1
  3/1 -> 2/2

== system mylib/278_dzt_v1/diff_trans_calc_H/simpcomp/orto_MUL_orto ==
  F1re : Inport
  F1im : Inport  Port=2
  F2re : Inport  Port=3
  F2im : Inport  Port=4
  1 : Sum  Inputs=+-
  {2..5} (4 alike) : Product
  6 : Sum
  Fre : Outport
  Fim : Outport  Port=2
  wires:
  F2re/1 -> 4/2, 2/2
  F1im/1 -> 3/1, 4/1
  F2im/1 -> 3/2, 5/2
  5/1 -> 6/2
  4/1 -> 6/1
  3/1 -> 1/2
  2/1 -> 1/1
  6/1 -> Fim/1
  1/1 -> Fre/1
  F1re/1 -> 2/1, 5/1

== system mylib/278_dzt_v1/diff_trans_calc_H/simpcomp/orto_MUL_orto1 ==
  F1re : Inport
  F1im : Inport  Port=2
  F2re : Inport  Port=3
  F2im : Inport  Port=4
  1 : Sum  Inputs=+-
  {2..5} (4 alike) : Product
  6 : Sum
  Fre : Outport
  Fim : Outport  Port=2
  wires:
  F2re/1 -> 4/2, 2/2
  F1im/1 -> 3/1, 4/1
  F2im/1 -> 3/2, 5/2
  5/1 -> 6/2
  4/1 -> 6/1
  3/1 -> 1/2
  2/1 -> 1/1
  6/1 -> Fim/1
  1/1 -> Fre/1
  F1re/1 -> 2/1, 5/1

== system mylib/278_dzt_v1/diff_trans_calc_H/simpcomp/orto_MUL_orto2 ==
  F1re : Inport
  F1im : Inport  Port=2
  F2re : Inport  Port=3
  F2im : Inport  Port=4
  1 : Sum  Inputs=+-
  {2..5} (4 alike) : Product
  6 : Sum
  Fre : Outport
  Fim : Outport  Port=2
  wires:
  F2re/1 -> 4/2, 2/2
  F1im/1 -> 3/1, 4/1
  F2im/1 -> 3/2, 5/2
  5/1 -> 6/2
  4/1 -> 6/1
  3/1 -> 1/2
  2/1 -> 1/1
  6/1 -> Fim/1
  1/1 -> Fre/1
  F1re/1 -> 2/1, 5/1

== system mylib/278_dzt_v1/diff_trans_calc_H/simpcomp/orto_MUL_orto3 ==
  F1re : Inport
  F1im : Inport  Port=2
  F2re : Inport  Port=3
  F2im : Inport  Port=4
  1 : Sum  Inputs=+-
  {2..5} (4 alike) : Product
  6 : Sum
  Fre : Outport
  Fim : Outport  Port=2
  wires:
  F2re/1 -> 4/2, 2/2
  F1im/1 -> 3/1, 4/1
  F2im/1 -> 3/2, 5/2
  5/1 -> 6/2
  4/1 -> 6/1
  3/1 -> 1/2
  2/1 -> 1/1
  6/1 -> Fim/1
  1/1 -> Fre/1
  F1re/1 -> 2/1, 5/1

== system mylib/278_dzt_v1/diff_trans_calc_H1/Ia_calc/orto_MUL_orto ==
  F1re : Inport
  F1im : Inport  Port=2
  F2re : Inport  Port=3
  F2im : Inport  Port=4
  1 : Sum  Inputs=+-
  {2..5} (4 alike) : Product
  6 : Sum
  Fre : Outport
  Fim : Outport  Port=2
  wires:
  F2re/1 -> 4/2, 2/2
  F1im/1 -> 3/1, 4/1
  F2im/1 -> 3/2, 5/2
  5/1 -> 6/2
  4/1 -> 6/1
  3/1 -> 1/2
  2/1 -> 1/1
  6/1 -> Fim/1
  1/1 -> Fre/1
  F1re/1 -> 2/1, 5/1

== system mylib/278_dzt_v1/diff_trans_calc_H1/Ia_calc/orto_to_arg ==
  re : Inport
  im : Inport  Port=2
  1 : Sum
  11 : Product  Inputs=*/  RndMeth=Zero  SaturateOnIntegerOverflow=on
  154 : Constant  Value=-1
  2 : Product
  3 : Switch  Criteria=u2 > Threshold
  4 : Sqrt  SaturateOnIntegerOverflow=on
  5 : Trigonometry  Operator=acos
  6 : Product
  7 : RelationalOperator  Operator=>  OutDataTypeStr=boolean  RndMeth=Simplest
  8 : Constant  Value=0
  9 : Product
  arg : Outport
  wires:
  4/1 -> 11/2
  11/1 -> 5/1
  2/1 -> 1/1
  6/1 -> 1/2
  1/1 -> 4/1
  5/1 -> 9/1, 3/1
  154/1 -> 9/2
  7/1 -> 3/2
  9/1 -> 3/3
  8/1 -> 7/2
  re/1 -> 2/1, 11/1, 2/2
  im/1 -> 6/1, 6/2, 7/1
  3/1 -> arg/1

== system mylib/278_dzt_v1/diff_trans_calc_H1/Ia_diff_calc/module1 ==
  Re : Inport
  Im : Inport  Port=2
  1 : Product  Inputs=**
  2 : Sum
  3 : Product  Inputs=**
  4 : Sqrt  SaturateOnIntegerOverflow=on
  Module : Outport
  wires:
  Re/1 -> 1/1, 1/2
  2/1 -> 4/1
  4/1 -> Module/1
  Im/1 -> 3/2, 3/1
  1/1 -> 2/1
  3/1 -> 2/2

== system mylib/278_dzt_v1/diff_trans_calc_H1/Ia_diff_calc/module2 ==
  Re : Inport
  Im : Inport  Port=2
  1 : Product  Inputs=**
  2 : Sum
  3 : Product  Inputs=**
  4 : Sqrt  SaturateOnIntegerOverflow=on
  Module : Outport
  wires:
  Re/1 -> 1/1, 1/2
  2/1 -> 4/1
  4/1 -> Module/1
  Im/1 -> 3/2, 3/1
  1/1 -> 2/1
  3/1 -> 2/2

== system mylib/278_dzt_v1/diff_trans_calc_H1/Ib_calc/orto_MUL_orto ==
  F1re : Inport
  F1im : Inport  Port=2
  F2re : Inport  Port=3
  F2im : Inport  Port=4
  1 : Sum  Inputs=+-
  {2..5} (4 alike) : Product
  6 : Sum
  Fre : Outport
  Fim : Outport  Port=2
  wires:
  F2re/1 -> 4/2, 2/2
  F1im/1 -> 3/1, 4/1
  F2im/1 -> 3/2, 5/2
  5/1 -> 6/2
  4/1 -> 6/1
  3/1 -> 1/2
  2/1 -> 1/1
  6/1 -> Fim/1
  1/1 -> Fre/1
  F1re/1 -> 2/1, 5/1

== system mylib/278_dzt_v1/diff_trans_calc_H1/Ib_calc/orto_to_arg ==
  re : Inport
  im : Inport  Port=2
  1 : Sum
  11 : Product  Inputs=*/  RndMeth=Zero  SaturateOnIntegerOverflow=on
  154 : Constant  Value=-1
  2 : Product
  3 : Switch  Criteria=u2 > Threshold
  4 : Sqrt  SaturateOnIntegerOverflow=on
  5 : Trigonometry  Operator=acos
  6 : Product
  7 : RelationalOperator  Operator=>  OutDataTypeStr=boolean  RndMeth=Simplest
  8 : Constant  Value=0
  9 : Product
  arg : Outport
  wires:
  4/1 -> 11/2
  11/1 -> 5/1
  2/1 -> 1/1
  6/1 -> 1/2
  1/1 -> 4/1
  5/1 -> 9/1, 3/1
  154/1 -> 9/2
  7/1 -> 3/2
  9/1 -> 3/3
  8/1 -> 7/2
  re/1 -> 2/1, 11/1, 2/2
  im/1 -> 6/1, 6/2, 7/1
  3/1 -> arg/1

== system mylib/278_dzt_v1/diff_trans_calc_H1/Ib_diff_calc/module1 ==
  Re : Inport
  Im : Inport  Port=2
  1 : Product  Inputs=**
  2 : Sum
  3 : Product  Inputs=**
  4 : Sqrt  SaturateOnIntegerOverflow=on
  Module : Outport
  wires:
  Re/1 -> 1/1, 1/2
  2/1 -> 4/1
  4/1 -> Module/1
  Im/1 -> 3/2, 3/1
  1/1 -> 2/1
  3/1 -> 2/2

== system mylib/278_dzt_v1/diff_trans_calc_H1/Ib_diff_calc/module2 ==
  Re : Inport
  Im : Inport  Port=2
  1 : Product  Inputs=**
  2 : Sum
  3 : Product  Inputs=**
  4 : Sqrt  SaturateOnIntegerOverflow=on
  Module : Outport
  wires:
  Re/1 -> 1/1, 1/2
  2/1 -> 4/1
  4/1 -> Module/1
  Im/1 -> 3/2, 3/1
  1/1 -> 2/1
  3/1 -> 2/2

== system mylib/278_dzt_v1/diff_trans_calc_H1/Ic_calc/orto_MUL_orto ==
  F1re : Inport
  F1im : Inport  Port=2
  F2re : Inport  Port=3
  F2im : Inport  Port=4
  1 : Sum  Inputs=+-
  {2..5} (4 alike) : Product
  6 : Sum
  Fre : Outport
  Fim : Outport  Port=2
  wires:
  F2re/1 -> 4/2, 2/2
  F1im/1 -> 3/1, 4/1
  F2im/1 -> 3/2, 5/2
  5/1 -> 6/2
  4/1 -> 6/1
  3/1 -> 1/2
  2/1 -> 1/1
  6/1 -> Fim/1
  1/1 -> Fre/1
  F1re/1 -> 2/1, 5/1

== system mylib/278_dzt_v1/diff_trans_calc_H1/Ic_calc/orto_to_arg ==
  re : Inport
  im : Inport  Port=2
  1 : Sum
  11 : Product  Inputs=*/  RndMeth=Zero  SaturateOnIntegerOverflow=on
  154 : Constant  Value=-1
  2 : Product
  3 : Switch  Criteria=u2 > Threshold
  4 : Sqrt  SaturateOnIntegerOverflow=on
  5 : Trigonometry  Operator=acos
  6 : Product
  7 : RelationalOperator  Operator=>  OutDataTypeStr=boolean  RndMeth=Simplest
  8 : Constant  Value=0
  9 : Product
  arg : Outport
  wires:
  4/1 -> 11/2
  11/1 -> 5/1
  2/1 -> 1/1
  6/1 -> 1/2
  1/1 -> 4/1
  5/1 -> 9/1, 3/1
  154/1 -> 9/2
  7/1 -> 3/2
  9/1 -> 3/3
  8/1 -> 7/2
  re/1 -> 2/1, 11/1, 2/2
  im/1 -> 6/1, 6/2, 7/1
  3/1 -> arg/1

== system mylib/278_dzt_v1/diff_trans_calc_H1/Ic_diff_calc/module1 ==
  Re : Inport
  Im : Inport  Port=2
  1 : Product  Inputs=**
  2 : Sum
  3 : Product  Inputs=**
  4 : Sqrt  SaturateOnIntegerOverflow=on
  Module : Outport
  wires:
  Re/1 -> 1/1, 1/2
  2/1 -> 4/1
  4/1 -> Module/1
  Im/1 -> 3/2, 3/1
  1/1 -> 2/1
  3/1 -> 2/2

== system mylib/278_dzt_v1/diff_trans_calc_H1/Ic_diff_calc/module2 ==
  Re : Inport
  Im : Inport  Port=2
  1 : Product  Inputs=**
  2 : Sum
  3 : Product  Inputs=**
  4 : Sqrt  SaturateOnIntegerOverflow=on
  Module : Outport
  wires:
  Re/1 -> 1/1, 1/2
  2/1 -> 4/1
  4/1 -> Module/1
  Im/1 -> 3/2, 3/1
  1/1 -> 2/1
  3/1 -> 2/2

== system mylib/278_dzt_v1/diff_trans_calc_H1/simpcomp/orto_MUL_orto ==
  F1re : Inport
  F1im : Inport  Port=2
  F2re : Inport  Port=3
  F2im : Inport  Port=4
  1 : Sum  Inputs=+-
  {2..5} (4 alike) : Product
  6 : Sum
  Fre : Outport
  Fim : Outport  Port=2
  wires:
  F2re/1 -> 4/2, 2/2
  F1im/1 -> 3/1, 4/1
  F2im/1 -> 3/2, 5/2
  5/1 -> 6/2
  4/1 -> 6/1
  3/1 -> 1/2
  2/1 -> 1/1
  6/1 -> Fim/1
  1/1 -> Fre/1
  F1re/1 -> 2/1, 5/1

== system mylib/278_dzt_v1/diff_trans_calc_H1/simpcomp/orto_MUL_orto1 ==
  F1re : Inport
  F1im : Inport  Port=2
  F2re : Inport  Port=3
  F2im : Inport  Port=4
  1 : Sum  Inputs=+-
  {2..5} (4 alike) : Product
  6 : Sum
  Fre : Outport
  Fim : Outport  Port=2
  wires:
  F2re/1 -> 4/2, 2/2
  F1im/1 -> 3/1, 4/1
  F2im/1 -> 3/2, 5/2
  5/1 -> 6/2
  4/1 -> 6/1
  3/1 -> 1/2
  2/1 -> 1/1
  6/1 -> Fim/1
  1/1 -> Fre/1
  F1re/1 -> 2/1, 5/1

== system mylib/278_dzt_v1/diff_trans_calc_H1/simpcomp/orto_MUL_orto2 ==
  F1re : Inport
  F1im : Inport  Port=2
  F2re : Inport  Port=3
  F2im : Inport  Port=4
  1 : Sum  Inputs=+-
  {2..5} (4 alike) : Product
  6 : Sum
  Fre : Outport
  Fim : Outport  Port=2
  wires:
  F2re/1 -> 4/2, 2/2
  F1im/1 -> 3/1, 4/1
  F2im/1 -> 3/2, 5/2
  5/1 -> 6/2
  4/1 -> 6/1
  3/1 -> 1/2
  2/1 -> 1/1
  6/1 -> Fim/1
  1/1 -> Fre/1
  F1re/1 -> 2/1, 5/1

== system mylib/278_dzt_v1/diff_trans_calc_H1/simpcomp/orto_MUL_orto3 ==
  F1re : Inport
  F1im : Inport  Port=2
  F2re : Inport  Port=3
  F2im : Inport  Port=4
  1 : Sum  Inputs=+-
  {2..5} (4 alike) : Product
  6 : Sum
  Fre : Outport
  Fim : Outport  Port=2
  wires:
  F2re/1 -> 4/2, 2/2
  F1im/1 -> 3/1, 4/1
  F2im/1 -> 3/2, 5/2
  5/1 -> 6/2
  4/1 -> 6/1
  3/1 -> 1/2
  2/1 -> 1/1
  6/1 -> Fim/1
  1/1 -> Fre/1
  F1re/1 -> 2/1, 5/1

== system mylib/278_dzt_v1/diff_trans_calc_H2/Ia_calc/orto_MUL_orto ==
  F1re : Inport
  F1im : Inport  Port=2
  F2re : Inport  Port=3
  F2im : Inport  Port=4
  1 : Sum  Inputs=+-
  {2..5} (4 alike) : Product
  6 : Sum
  Fre : Outport
  Fim : Outport  Port=2
  wires:
  F2re/1 -> 4/2, 2/2
  F1im/1 -> 3/1, 4/1
  F2im/1 -> 3/2, 5/2
  5/1 -> 6/2
  4/1 -> 6/1
  3/1 -> 1/2
  2/1 -> 1/1
  6/1 -> Fim/1
  1/1 -> Fre/1
  F1re/1 -> 2/1, 5/1

== system mylib/278_dzt_v1/diff_trans_calc_H2/Ia_calc/orto_to_arg ==
  re : Inport
  im : Inport  Port=2
  1 : Sum
  11 : Product  Inputs=*/  RndMeth=Zero  SaturateOnIntegerOverflow=on
  154 : Constant  Value=-1
  2 : Product
  3 : Switch  Criteria=u2 > Threshold
  4 : Sqrt  SaturateOnIntegerOverflow=on
  5 : Trigonometry  Operator=acos
  6 : Product
  7 : RelationalOperator  Operator=>  OutDataTypeStr=boolean  RndMeth=Simplest
  8 : Constant  Value=0
  9 : Product
  arg : Outport
  wires:
  4/1 -> 11/2
  11/1 -> 5/1
  2/1 -> 1/1
  6/1 -> 1/2
  1/1 -> 4/1
  5/1 -> 9/1, 3/1
  154/1 -> 9/2
  7/1 -> 3/2
  9/1 -> 3/3
  8/1 -> 7/2
  re/1 -> 2/1, 11/1, 2/2
  im/1 -> 6/1, 6/2, 7/1
  3/1 -> arg/1

== system mylib/278_dzt_v1/diff_trans_calc_H2/Ia_diff_calc/module1 ==
  Re : Inport
  Im : Inport  Port=2
  1 : Product  Inputs=**
  2 : Sum
  3 : Product  Inputs=**
  4 : Sqrt  SaturateOnIntegerOverflow=on
  Module : Outport
  wires:
  Re/1 -> 1/1, 1/2
  2/1 -> 4/1
  4/1 -> Module/1
  Im/1 -> 3/2, 3/1
  1/1 -> 2/1
  3/1 -> 2/2

== system mylib/278_dzt_v1/diff_trans_calc_H2/Ia_diff_calc/module2 ==
  Re : Inport
  Im : Inport  Port=2
  1 : Product  Inputs=**
  2 : Sum
  3 : Product  Inputs=**
  4 : Sqrt  SaturateOnIntegerOverflow=on
  Module : Outport
  wires:
  Re/1 -> 1/1, 1/2
  2/1 -> 4/1
  4/1 -> Module/1
  Im/1 -> 3/2, 3/1
  1/1 -> 2/1
  3/1 -> 2/2

== system mylib/278_dzt_v1/diff_trans_calc_H2/Ib_calc/orto_MUL_orto ==
  F1re : Inport
  F1im : Inport  Port=2
  F2re : Inport  Port=3
  F2im : Inport  Port=4
  1 : Sum  Inputs=+-
  {2..5} (4 alike) : Product
  6 : Sum
  Fre : Outport
  Fim : Outport  Port=2
  wires:
  F2re/1 -> 4/2, 2/2
  F1im/1 -> 3/1, 4/1
  F2im/1 -> 3/2, 5/2
  5/1 -> 6/2
  4/1 -> 6/1
  3/1 -> 1/2
  2/1 -> 1/1
  6/1 -> Fim/1
  1/1 -> Fre/1
  F1re/1 -> 2/1, 5/1

== system mylib/278_dzt_v1/diff_trans_calc_H2/Ib_calc/orto_to_arg ==
  re : Inport
  im : Inport  Port=2
  1 : Sum
  11 : Product  Inputs=*/  RndMeth=Zero  SaturateOnIntegerOverflow=on
  154 : Constant  Value=-1
  2 : Product
  3 : Switch  Criteria=u2 > Threshold
  4 : Sqrt  SaturateOnIntegerOverflow=on
  5 : Trigonometry  Operator=acos
  6 : Product
  7 : RelationalOperator  Operator=>  OutDataTypeStr=boolean  RndMeth=Simplest
  8 : Constant  Value=0
  9 : Product
  arg : Outport
  wires:
  4/1 -> 11/2
  11/1 -> 5/1
  2/1 -> 1/1
  6/1 -> 1/2
  1/1 -> 4/1
  5/1 -> 9/1, 3/1
  154/1 -> 9/2
  7/1 -> 3/2
  9/1 -> 3/3
  8/1 -> 7/2
  re/1 -> 2/1, 11/1, 2/2
  im/1 -> 6/1, 6/2, 7/1
  3/1 -> arg/1

== system mylib/278_dzt_v1/diff_trans_calc_H2/Ib_diff_calc/module1 ==
  Re : Inport
  Im : Inport  Port=2
  1 : Product  Inputs=**
  2 : Sum
  3 : Product  Inputs=**
  4 : Sqrt  SaturateOnIntegerOverflow=on
  Module : Outport
  wires:
  Re/1 -> 1/1, 1/2
  2/1 -> 4/1
  4/1 -> Module/1
  Im/1 -> 3/2, 3/1
  1/1 -> 2/1
  3/1 -> 2/2

== system mylib/278_dzt_v1/diff_trans_calc_H2/Ib_diff_calc/module2 ==
  Re : Inport
  Im : Inport  Port=2
  1 : Product  Inputs=**
  2 : Sum
  3 : Product  Inputs=**
  4 : Sqrt  SaturateOnIntegerOverflow=on
  Module : Outport
  wires:
  Re/1 -> 1/1, 1/2
  2/1 -> 4/1
  4/1 -> Module/1
  Im/1 -> 3/2, 3/1
  1/1 -> 2/1
  3/1 -> 2/2

== system mylib/278_dzt_v1/diff_trans_calc_H2/Ic_calc/orto_MUL_orto ==
  F1re : Inport
  F1im : Inport  Port=2
  F2re : Inport  Port=3
  F2im : Inport  Port=4
  1 : Sum  Inputs=+-
  {2..5} (4 alike) : Product
  6 : Sum
  Fre : Outport
  Fim : Outport  Port=2
  wires:
  F2re/1 -> 4/2, 2/2
  F1im/1 -> 3/1, 4/1
  F2im/1 -> 3/2, 5/2
  5/1 -> 6/2
  4/1 -> 6/1
  3/1 -> 1/2
  2/1 -> 1/1
  6/1 -> Fim/1
  1/1 -> Fre/1
  F1re/1 -> 2/1, 5/1

== system mylib/278_dzt_v1/diff_trans_calc_H2/Ic_calc/orto_to_arg ==
  re : Inport
  im : Inport  Port=2
  1 : Sum
  11 : Product  Inputs=*/  RndMeth=Zero  SaturateOnIntegerOverflow=on
  154 : Constant  Value=-1
  2 : Product
  3 : Switch  Criteria=u2 > Threshold
  4 : Sqrt  SaturateOnIntegerOverflow=on
  5 : Trigonometry  Operator=acos
  6 : Product
  7 : RelationalOperator  Operator=>  OutDataTypeStr=boolean  RndMeth=Simplest
  8 : Constant  Value=0
  9 : Product
  arg : Outport
  wires:
  4/1 -> 11/2
  11/1 -> 5/1
  2/1 -> 1/1
  6/1 -> 1/2
  1/1 -> 4/1
  5/1 -> 9/1, 3/1
  154/1 -> 9/2
  7/1 -> 3/2
  9/1 -> 3/3
  8/1 -> 7/2
  re/1 -> 2/1, 11/1, 2/2
  im/1 -> 6/1, 6/2, 7/1
  3/1 -> arg/1

== system mylib/278_dzt_v1/diff_trans_calc_H2/Ic_diff_calc/module1 ==
  Re : Inport
  Im : Inport  Port=2
  1 : Product  Inputs=**
  2 : Sum
  3 : Product  Inputs=**
  4 : Sqrt  SaturateOnIntegerOverflow=on
  Module : Outport
  wires:
  Re/1 -> 1/1, 1/2
  2/1 -> 4/1
  4/1 -> Module/1
  Im/1 -> 3/2, 3/1
  1/1 -> 2/1
  3/1 -> 2/2

== system mylib/278_dzt_v1/diff_trans_calc_H2/Ic_diff_calc/module2 ==
  Re : Inport
  Im : Inport  Port=2
  1 : Product  Inputs=**
  2 : Sum
  3 : Product  Inputs=**
  4 : Sqrt  SaturateOnIntegerOverflow=on
  Module : Outport
  wires:
  Re/1 -> 1/1, 1/2
  2/1 -> 4/1
  4/1 -> Module/1
  Im/1 -> 3/2, 3/1
  1/1 -> 2/1
  3/1 -> 2/2

== system mylib/278_dzt_v1/diff_trans_calc_H2/simpcomp/orto_MUL_orto ==
  F1re : Inport
  F1im : Inport  Port=2
  F2re : Inport  Port=3
  F2im : Inport  Port=4
  1 : Sum  Inputs=+-
  {2..5} (4 alike) : Product
  6 : Sum
  Fre : Outport
  Fim : Outport  Port=2
  wires:
  F2re/1 -> 4/2, 2/2
  F1im/1 -> 3/1, 4/1
  F2im/1 -> 3/2, 5/2
  5/1 -> 6/2
  4/1 -> 6/1
  3/1 -> 1/2
  2/1 -> 1/1
  6/1 -> Fim/1
  1/1 -> Fre/1
  F1re/1 -> 2/1, 5/1

== system mylib/278_dzt_v1/diff_trans_calc_H2/simpcomp/orto_MUL_orto1 ==
  F1re : Inport
  F1im : Inport  Port=2
  F2re : Inport  Port=3
  F2im : Inport  Port=4
  1 : Sum  Inputs=+-
  {2..5} (4 alike) : Product
  6 : Sum
  Fre : Outport
  Fim : Outport  Port=2
  wires:
  F2re/1 -> 4/2, 2/2
  F1im/1 -> 3/1, 4/1
  F2im/1 -> 3/2, 5/2
  5/1 -> 6/2
  4/1 -> 6/1
  3/1 -> 1/2
  2/1 -> 1/1
  6/1 -> Fim/1
  1/1 -> Fre/1
  F1re/1 -> 2/1, 5/1

== system mylib/278_dzt_v1/diff_trans_calc_H2/simpcomp/orto_MUL_orto2 ==
  F1re : Inport
  F1im : Inport  Port=2
  F2re : Inport  Port=3
  F2im : Inport  Port=4
  1 : Sum  Inputs=+-
  {2..5} (4 alike) : Product
  6 : Sum
  Fre : Outport
  Fim : Outport  Port=2
  wires:
  F2re/1 -> 4/2, 2/2
  F1im/1 -> 3/1, 4/1
  F2im/1 -> 3/2, 5/2
  5/1 -> 6/2
  4/1 -> 6/1
  3/1 -> 1/2
  2/1 -> 1/1
  6/1 -> Fim/1
  1/1 -> Fre/1
  F1re/1 -> 2/1, 5/1

== system mylib/278_dzt_v1/diff_trans_calc_H2/simpcomp/orto_MUL_orto3 ==
  F1re : Inport
  F1im : Inport  Port=2
  F2re : Inport  Port=3
  F2im : Inport  Port=4
  1 : Sum  Inputs=+-
  {2..5} (4 alike) : Product
  6 : Sum
  Fre : Outport
  Fim : Outport  Port=2
  wires:
  F2re/1 -> 4/2, 2/2
  F1im/1 -> 3/1, 4/1
  F2im/1 -> 3/2, 5/2
  5/1 -> 6/2
  4/1 -> 6/1
  3/1 -> 1/2
  2/1 -> 1/1
  6/1 -> Fim/1
  1/1 -> Fre/1
  F1re/1 -> 2/1, 5/1

== system mylib/Inverse time-delay/ANSI Inverse time-delay/Equation ANSI/Zero_check ==
  in : Inport
  Constant : Constant  Value=0
  Constant1 : Constant  Value=0.000001
  Relational Operator : RelationalOperator  Operator===  OutDataTypeStr=boolean  RndMeth=Simplest
  Switch : Switch  Criteria=u2 > Threshold
  out : Outport
  wires:
  in/1 -> Switch/3, Relational Operator/1
  Constant/1 -> Relational Operator/2
  Relational Operator/1 -> Switch/2
  Constant1/1 -> Switch/1
  Switch/1 -> out/1

== system mylib/Inverse time-delay/ANSI Inverse time-delay/Equation ANSI/Zero_check1 ==
  in : Inport
  Constant : Constant  Value=0
  Constant1 : Constant  Value=0.000001
  Relational Operator : RelationalOperator  Operator===  OutDataTypeStr=boolean  RndMeth=Simplest
  Switch : Switch  Criteria=u2 > Threshold
  out : Outport
  wires:
  in/1 -> Switch/3, Relational Operator/1
  Constant/1 -> Relational Operator/2
  Relational Operator/1 -> Switch/2
  Constant1/1 -> Switch/1
  Switch/1 -> out/1

== system mylib/Inverse time-delay/ANSI Inverse time-delay inductive disk relay/Equation ANSI_idr/Zero_check ==
  in : Inport
  Constant : Constant  Value=0
  Constant1 : Constant  Value=0.000001
  Relational Operator : RelationalOperator  Operator===  OutDataTypeStr=boolean  RndMeth=Simplest
  Switch : Switch  Criteria=u2 > Threshold
  out : Outport
  wires:
  in/1 -> Switch/3, Relational Operator/1
  Constant/1 -> Relational Operator/2
  Relational Operator/1 -> Switch/2
  Constant1/1 -> Switch/1
  Switch/1 -> out/1

== system mylib/Inverse time-delay/ANSI Inverse time-delay inductive disk relay/Equation ANSI_idr/Zero_check1 ==
  in : Inport
  Constant : Constant  Value=0
  Constant1 : Constant  Value=0.000001
  Relational Operator : RelationalOperator  Operator===  OutDataTypeStr=boolean  RndMeth=Simplest
  Switch : Switch  Criteria=u2 > Threshold
  out : Outport
  wires:
  in/1 -> Switch/3, Relational Operator/1
  Constant/1 -> Relational Operator/2
  Relational Operator/1 -> Switch/2
  Constant1/1 -> Switch/1
  Switch/1 -> out/1
